simulink model "sim_kinematic_control"  (R2018a)
settings: Solver=ode3  StartTime=0.0  StopTime=10  FixedStep=0.02  RelTol=1e-3
settings Model: Creator=E183308  LastModifiedBy=E183308

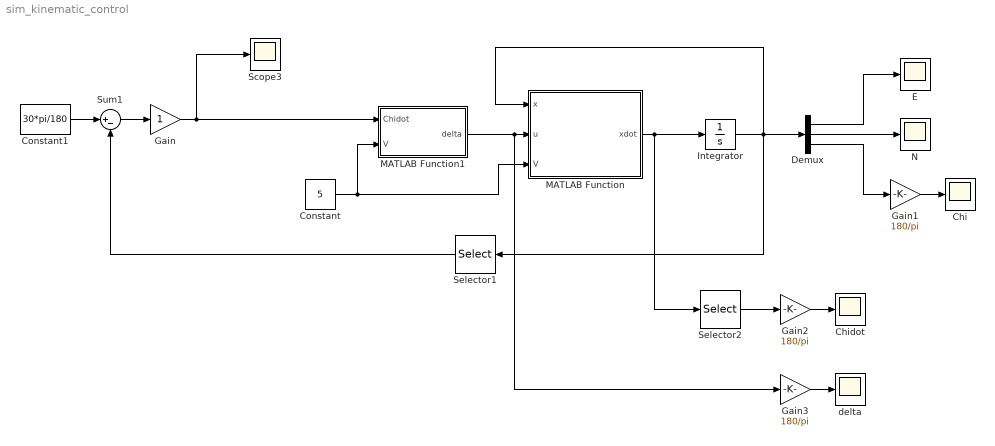
== system sim_kinematic_control ==
  Chi : Scope
  Chidot : Scope
  Constant : Constant  Value=5
  Constant1 : Constant  Value=30*pi/180
  Demux : Demux  Outputs=3
  E : Scope
  Gain : Gain
  Gain1 : Gain  Gain=180/pi
  Gain2 : Gain  Gain=180/pi
  Gain3 : Gain  Gain=180/pi
  Integrator : Integrator  InitialCondition=[0;0;0]
  MATLAB Function : MATLAB Function  TreatAsAtomicUnit=on
  MATLAB Function1 : MATLAB Function  TreatAsAtomicUnit=on
  N : Scope
  Scope3 : Scope
  Selector1 : Selector  InputPortWidth=3  IndexOptions=Index vector (dialog)  Indices=3  OutputSizes=1
  Selector2 : Selector  InputPortWidth=3  IndexOptions=Index vector (dialog)  Indices=3  OutputSizes=1
  Sum1 : Sum  Inputs=|+-
  delta : Scope
  wires:
  Sum1/1 -> Gain/1
  Selector1/1 -> Sum1/2
  Constant/1 -> MATLAB Function1/2(V), MATLAB Function/3(V)
  MATLAB Function/1(xdot) -> Selector2/1, Integrator/1
  Gain/1 -> MATLAB Function1/1(Chidot), Scope3/1
  Demux/1 -> E/1
  Demux/2 -> N/1
  Demux/3 -> Gain1/1
  Gain1/1 -> Chi/1
  Integrator/1 -> Selector1/1, MATLAB Function/1(x), Demux/1
  MATLAB Function1/1(delta) -> Gain3/1, MATLAB Function/2(u)
  Constant1/1 -> Sum1/1
  Gain2/1 -> Chidot/1
  Selector2/1 -> Gain2/1
  Gain3/1 -> delta/1

== matlab function sim_kinematic_control/MATLAB Function1 ==
  data: Chidot input; delta output; V input
function delta = fcn(Chidot,V)

L = 10; % ft

if abs(V) > 0
    delta = atan2(L*Chidot,V);
else
    delta = 0;
end

== matlab function sim_kinematic_control/MATLAB Function ==
  data: x input; u input; xdot output; V input
function xdot = kinematic(x,u,V)

L = 10; % ft

E = x(1);
N = x(2);
Chi = x(3);

delta = u;

Edot = V*sin(Chi);
Ndot = V*cos(Chi);
Chidot = V/L*tan(delta);

xdot = [Edot; Ndot; Chidot];
